simulink model "untitled1"  (R2024a)
settings: Solver=VariableStepAuto  StartTime=0.0  StopTime=10.0  RelTol=1e-3
undefined symbols (not defined in the file): pathXY, route1_waypoint_raw, route2_waypoint_raw, route3_waypoint_raw
libraries: CarMaker4SL x96, slpidlib x2
(part 3 of 3)

== matlab function untitled1/Final Project1/Scenario 1/MATLAB Function1 ==
  settings: updateMethod=DISCRETE  sampleTime=0.05
  data: s_ref input; path output; obs input; mapx input; mapy input; opt_ind output; x output; path1 output; opt_ind1 output; y output
function [path,opt_ind, x, path1,opt_ind1, y] = trajectory_path(s_ref, obs, mapx, mapy)

    % Frenet 상태 초기화
    si = s0;
    si_d = v0 * cos(yawi);
    si_dd = a0 * cos(yawi);
    sf_d = 1.0; sf_dd = 0;

    di = d0;
    di_d = v0 * sin(yawi);
    di_dd = a0 * sin(yawi);
    df_d = 0; df_dd = 0;

    si    = path(opt_ind).s(7);
    si_d  = path(opt_ind).s_d(7);
    si_dd = path(opt_ind).s_dd(7);

    di    = path(opt_ind).d(7);
    di_d  = path(opt_ind).d_d(7);
    di_dd = path(opt_ind).d_dd(7);

    opt_d = path(opt_ind).d(end);  % 일관성 유지용

end
function [path, opt_ind] = frenet_optimal_planning(si, si_d, si_dd, ...
                                              sf_d, sf_dd, di, di_d, di_dd, df_d, df_dd, ...
                                              obs, mapx, mapy, s_ref, opt_d)
    
end
    global K_J K_T K_D K_V W_LAT W_LON
    % K_J Jerk 웨이트 s,d 둘다 , K_T t_f에 대한 항, K_D Diff d에대한 diff, K_V s에 대한 diff(속도 s_d에 대한 diff)

    K_J = 0.1; K_T = 1; K_D = 1; K_V = 1;

    W_LAT = 1.0; W_LON = 1.0; %종방향 횡방향 웨이트

    global fp_templet
    fp_templet= struct( ...
    't', [], 'd', 0, 'd_d', 0, 'd_dd', 0, 'd_ddd', 0, ...
    's', 0, 's_d', 0, 's_dd', 0, 's_ddd', 0, ...
    'c_lat', 0, 'c_lon', 0, 'c_tot', 0, ...
    'x', [], 'y', [], 'yaw', [], 'ds', [], 'kappa', []);


    % 1. Frenet 궤적 후보 생성
    fplist = calc_frenet_paths(si, si_d, si_dd, sf_d, sf_dd, di, di_d, di_dd, df_d, df_dd, opt_d);

    % 2. Global 궤적 변환
    fplist = calc_global_paths(fplist, mapx, mapy, s_ref);

    % 3. 제약조건 및 충돌 검사
    fplist = check_path(fplist, obs, mapx, mapy, s_ref);

    % 4. 최적 경로 선택
    min_cost = inf;
    opt_ind = 1;  % 초기값
    for i = 1:length(fplist)
        if fplist(i).c_tot < min_cost
            min_cost = fplist(i).c_tot;
            opt_ind = i;
        end
    end

    % 5. 출력
    path = fplist; 
end

function fplist = calc_frenet_paths(si, si_d, si_dd, sf_d, sf_dd, di, di_d, di_dd, df_d, df_dd, opt_d)
    global K_J K_T K_D K_V W_LAT W_LON TARGET_SPEED MIN_T MAX_T DT_T DT DF_SET fp_templet
    TARGET_SPEED=20;
    DF_SET = linspace(-3, 3, 3); 
    DT = 0.2; 
    DT_T = 0.5; 
    MIN_T = 11.0; 
    MAX_T = 14.0; 
    
    fplist = repmat(fp_templet, 1, 0);  % 빈 구조체 배열로 초기화
    fp=fp_templet;
    for df = DF_SET
        for T = MIN_T:DT_T:MAX_T
            fp=fp_templet;
            % Lateral trajectory (Quintic)
            [a0_d, a1_d, a2_d, a3_d, a4_d, a5_d] = calc_quintic(di, di_d, di_dd, df, df_d, df_dd, T);
            
            t = 0:DT:T;
     
            d = a0_d + a1_d*t + a2_d*t.^2 + a3_d*t.^3 + a4_d*t.^4 + a5_d*t.^5;
            d_d = a1_d + 2*a2_d*t + 3*a3_d*t.^2 + 4*a4_d*t.^3 + 5*a5_d*t.^4;
            d_dd = 2*a2_d + 6*a3_d*t + 12*a4_d*t.^2 + 20*a5_d*t.^3;
            d_ddd = 6*a3_d + 24*a4_d*t + 60*a5_d*t.^2;
            
            
            % Longitudinal trajectory (Quartic)
            %sf_d에 Target Speed를 기준으로 여러개 생성해야된다
            %sf 인자는 어디로 갔나
            [a0_s, a1_s, a2_s, a3_s, a4_s] = calc_quartic(si, si_d, si_dd, sf_d, sf_dd, T);
            s = a0_s + a1_s*t + a2_s*t.^2 + a3_s*t.^3 + a4_s*t.^4;
            s_d = a1_s + 2*a2_s*t + 3*a3_s*t.^2 + 4*a4_s*t.^3;
            s_dd = 2*a2_s + 6*a3_s*t + 12*a4_s*t.^2;
            s_ddd = 6*a3_s + 24*a4_s*t;
            
           
            %% 비용 계산
            J_lat = sum(d_ddd.^2); %적분항 인데 왜 T로 안나눠 임마 
            J_lon = sum(s_ddd.^2); %적분항 
            d_diff = (d(end) - opt_d)^2;  %차선변경 최소화
            s_diff = (TARGET_SPEED - s_d(end))^2; %ACC랑 최대한 유지하기 위함
            
            %% 비용함수
            c_lat = K_J * J_lat  + K_D * d_diff + K_T * T; %% cost_lateral
            c_lon = K_J * J_lon  + K_V * s_diff + K_T * T; %% cost_longitual
            c_tot = W_LAT * c_lat + W_LON * c_lon; %% total Cost가 낮은것을 선택 

            fp = struct('t', t, 'd', d, 'd_d', d_d, 'd_dd', d_dd, 'd_ddd', d_ddd, ...
            's', s, 's_d', s_d, 's_dd', s_dd, 's_ddd', s_ddd, ...
            'c_lat', c_lat, 'c_lon', c_lon, 'c_tot', c_tot, ...
            'x', [], 'y', [], 'yaw', [], 'ds', [], 'kappa', []);

            fplist(end+1) = fp;
        end 
    end
end

function fplist = calc_global_paths(fplist, mapx, mapy, s_ref)
    for i = 1:length(fplist)
        fp = fplist(i);
        fp.x = zeros(size(fp.s));
        fp.y = zeros(size(fp.s));
        fp.yaw = zeros(size(fp.s));
        fp.ds = zeros(size(fp.s)); % 곡률계산을 변환을 위해 
        fp.kappa = zeros(size(fp.s)); 

        for j = 1:length(fp.s)
            [fp.x(j), fp.y(j), ~] = get_cartesian(fp.s(j), fp.d(j), mapx, mapy, s_ref);
        end

        for j = 1:length(fp.x)-1
            dx = fp.x(j+1) - fp.x(j);
            dy = fp.y(j+1) - fp.y(j);
            fp.yaw(j) = atan2(dy, dx);
            fp.ds(j) = hypot(dx, dy);
        end
        fp.yaw(end) = fp.yaw(end-1);
        fp.ds(end) = fp.ds(end-1);

        for j = 1:length(fp.yaw)-1
            dyaw = atan2(sin(fp.yaw(j+1) - fp.yaw(j)), cos(fp.yaw(j+1) - fp.yaw(j)));
            fp.kappa(j) = dyaw / fp.ds(j);
        end
        fp.kappa(end) = fp.kappa(end-1);

        fplist(i) = fp;
    end
end


function fplist = check_path(fplist, obs, mapx, mapy, s_ref)
    global V_MAX ACC_MAX K_MAX COL_CHECK fp_templet
    V_MAX = 10;
    ACC_MAX=10;
    K_MAX=4; %
    COL_CHECK=0.25;
    valid_paths = repmat(fp_templet, 1, 0);  % 빈 구조체 배열로 초기화
   

    for i = 1:length(fplist)
        fp = fplist(i);
        acc_squared = fp.s_dd.^2 + fp.d_dd.^2;

        if all(fp.s_d) > V_MAX
            continue;
        elseif any(acc_squared > ACC_MAX^2)
            continue;
        elseif any(abs(fp.kappa) > K_MAX)
            continue;
        elseif collision_check(fp, obs, mapx, mapy, s_ref)
            continue;
        else
            valid_paths(end+1) = fp; 
        end
    end

    fplist = valid_paths;
end

function collision = collision_check(fp, obs, mapx, mapy, s_ref)
    
    CAR_RADIUS = 2;
    OBSTACLE_RADIUS = 0.5;
    SAFE_DIST = CAR_RADIUS + OBSTACLE_RADIUS;

    collision = false;
    for i = 1:size(obs,1)
        [x_obs, y_obs, ~] = get_cartesian(obs(i,1), obs(i,2), mapx, mapy, s_ref);
        dists = (fp.x - x_obs).^2 + (fp.y - y_obs).^2;
        if any(dists <= SAFE_DIST^2)
            collision = true;
            return;
        end
    end
end
